simulink model "RC_Circuit"  (R2020a)
settings: Solver=VariableStepAuto  StartTime=0.0  StopTime=10.0  RelTol=1e-3
PostLoadFcn:
  | R=10;
  | C=10*10^-6;
settings Model: Creator=NIKITA  LastModifiedBy=NIKITA

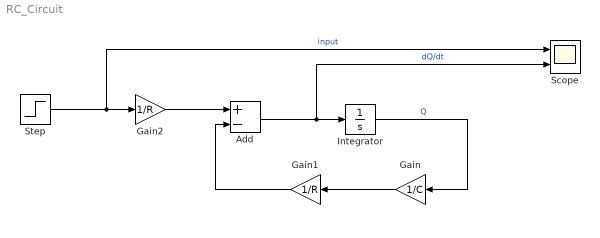
== system RC_Circuit ==
  Add : Sum  Inputs=+-
  Gain : Gain  Gain=1/C
  Gain1 : Gain  Gain=1/R
  Gain2 : Gain  Gain=1/R
  Integrator : Integrator
  Scope : Scope  NumInputPorts=2
  Step : Step  SampleTime=0
  wires:
  Add/1 -> Scope/2, Integrator/1  "dQ/dt"
  Integrator/1 -> Gain/1  "Q"
  Gain/1 -> Gain1/1
  Gain1/1 -> Add/2
  Gain2/1 -> Add/1
  Step/1 -> Scope/1, Gain2/1  "input"
